simulink model "xEMU_SimulationModel3_rule1"  (R2017b)
settings: Solver=ode4  StartTime=0.0  StopTime=8192  FixedStep=0.01  RelTol=1e-3
undefined symbols (not defined in the file): a1, a2, a3, a4, ACO, BAT, Battery, DCT, DRT, EMS, ENV, Fahrzyklus_VS_modell, height_BAT, leistung, lib_bat, Maximum, Maximum_position, Num_cells, P_FC_max_long, P_FC_min_long, P_FC_step_max, Pbat_charge_max, Pbat_discharge_max, Pfc_max, Pfc_min, SOC_tar, time_peaks, TRM, velocity_peaks
libraries: simulink x5
(part 4 of 15)

== system xEMU_SimulationModel3_rule1/Battery (BAT)_komplex/Subsystem/ElectricalCircuit/Cellelement_Elem1 ==
  OhmicResistance_Elem1 : Subsystem
  ParallelRC_Elem5 : Subsystem
  ParallelRC_Elem6 : Subsystem
  Rmphn_Elem2 : Subsystem
  Rmphn_Elem3 : Subsystem
  SoC : Integrator  InitialCondition=SOC_tar*100  LimitOutput=on  UpperSaturationLimit=100  LowerSaturationLimit=0
  SoCFactor : Gain  Gain=0.001207729468599
  SphericalDiffusion_Elem4 : Subsystem
  VoltageSource_Elem7 : Subsystem
  Out1 : Outport
  wires:
  [I_CellElement1] -> SoCFactor/1
  SoCFactor/1 -> SoC/1
  [T_CellElement1] -> ParallelRC_Elem6/1(T), VoltageSource_Elem7/1(T), ParallelRC_Elem5/1(T), SphericalDiffusion_Elem4/1(T), Rmphn_Elem3/1(T), Rmphn_Elem2/1(T), OhmicResistance_Elem1/1(T)
  SoC/1 -> Out1/1, ParallelRC_Elem6/2(SoC), VoltageSource_Elem7/2(SoC), ParallelRC_Elem5/2(SoC), SphericalDiffusion_Elem4/2(SoC), Rmphn_Elem3/2(SoC), Rmphn_Elem2/2(SoC), OhmicResistance_Elem1/2(SoC)

== system xEMU_SimulationModel3_rule1/Battery (BAT)_komplex/Subsystem/MatrixAxC/StateComponent0 ==
  Add5_1 : Sum
  ColConst : Constant  Value=0
  Const1_1 : Constant  Value=-1.000000
  Const1_5 : Constant  Value=0.991746
  Const1_6 : Constant  Value=0.991451
  Const2_2 : Constant  Value=0.991451
  Div2_1 : Product  Inputs=*/
  Div2_3 : Product  Inputs=*/
  Div2_4 : Product  Inputs=*/
  Div3_2 : Product  Inputs=*/
  Integrator : Integrator
  Mul3_4 : Product
  Mul4_1 : Product
  Mul4_2 : Product
  RowConst : Constant  Value=0
  Row : Outport
  Col : Outport  Port=2
  tag scope: State1=global
  wires:
  Integrator/1 -> [State1]
  ColConst/1 -> Col/1
  RowConst/1 -> Row/1
  Add5_1/1 -> Integrator/1
  Mul4_1/1 -> Add5_1/1
  [State1] -> Mul4_1/1
  Div3_2/1 -> Mul4_1/2
  Div2_1/1 -> Div3_2/1
  Const1_1/1 -> Div2_1/1
  [ID6_ObjTau] -> Div2_1/2
  Const2_2/1 -> Div3_2/2
  Mul4_2/1 -> Add5_1/2
  [InputCurrent] -> Mul4_2/1
  Mul3_4/1 -> Mul4_2/2
  Div2_3/1 -> Mul3_4/1
  [ID6_ObjR] -> Div2_3/1
  [ID6_ObjTau] -> Div2_3/2
  Div2_4/1 -> Mul3_4/2
  Const1_5/1 -> Div2_4/1
  Const1_6/1 -> Div2_4/2

== system xEMU_SimulationModel3_rule1/Battery (BAT)_komplex/Subsystem/MatrixAxC/StateComponent1 ==
  Add5_1 : Sum
  ColConst : Constant  Value=0
  Const1_1 : Constant  Value=-1.000000
  Const1_5 : Constant  Value=0.335190
  Const1_6 : Constant  Value=0.335870
  Const2_2 : Constant  Value=0.335870
  Div2_1 : Product  Inputs=*/
  Div2_3 : Product  Inputs=*/
  Div2_4 : Product  Inputs=*/
  Div3_2 : Product  Inputs=*/
  Integrator : Integrator
  Mul3_4 : Product
  Mul4_1 : Product
  Mul4_2 : Product
  RowConst : Constant
  Row : Outport
  Col : Outport  Port=2
  tag scope: State2=global
  wires:
  Integrator/1 -> [State2]
  ColConst/1 -> Col/1
  RowConst/1 -> Row/1
  Add5_1/1 -> Integrator/1
  Mul4_1/1 -> Add5_1/1
  [State2] -> Mul4_1/1
  Div3_2/1 -> Mul4_1/2
  Div2_1/1 -> Div3_2/1
  Const1_1/1 -> Div2_1/1
  [ID6_ObjTau] -> Div2_1/2
  Const2_2/1 -> Div3_2/2
  Mul4_2/1 -> Add5_1/2
  [InputCurrent] -> Mul4_2/1
  Mul3_4/1 -> Mul4_2/2
  Div2_3/1 -> Mul3_4/1
  [ID6_ObjR] -> Div2_3/1
  [ID6_ObjTau] -> Div2_3/2
  Div2_4/1 -> Mul3_4/2
  Const1_5/1 -> Div2_4/1
  Const1_6/1 -> Div2_4/2

== system xEMU_SimulationModel3_rule1/Battery (BAT)_komplex/Subsystem/MatrixAxC/StateComponent10 ==
  Add5_1 : Sum
  ColConst : Constant  Value=0
  Const1_1 : Constant  Value=-1.000000
  Const1_5 : Constant  Value=0.020606
  Const1_6 : Constant  Value=0.004354
  Const2_2 : Constant  Value=0.004354
  Div2_1 : Product  Inputs=*/
  Div2_3 : Product  Inputs=*/
  Div2_4 : Product  Inputs=*/
  Div3_2 : Product  Inputs=*/
  Integrator : Integrator
  Mul3_4 : Product
  Mul4_1 : Product
  Mul4_2 : Product
  RowConst : Constant  Value=10
  Row : Outport
  Col : Outport  Port=2
  tag scope: State11=global
  wires:
  Integrator/1 -> [State11]
  ColConst/1 -> Col/1
  RowConst/1 -> Row/1
  Add5_1/1 -> Integrator/1
  Mul4_1/1 -> Add5_1/1
  [State11] -> Mul4_1/1
  Div3_2/1 -> Mul4_1/2
  Div2_1/1 -> Div3_2/1
  Const1_1/1 -> Div2_1/1
  [ID6_ObjTau] -> Div2_1/2
  Const2_2/1 -> Div3_2/2
  Mul4_2/1 -> Add5_1/2
  [InputCurrent] -> Mul4_2/1
  Mul3_4/1 -> Mul4_2/2
  Div2_3/1 -> Mul3_4/1
  [ID6_ObjR] -> Div2_3/1
  [ID6_ObjTau] -> Div2_3/2
  Div2_4/1 -> Mul3_4/2
  Const1_5/1 -> Div2_4/1
  Const1_6/1 -> Div2_4/2

== system xEMU_SimulationModel3_rule1/Battery (BAT)_komplex/Subsystem/MatrixAxC/StateComponent11 ==
  Add5_1 : Sum
  ColConst : Constant  Value=0
  Const1_1 : Constant  Value=-1.000000
  Const1_5 : Constant  Value=0.016393
  Const1_6 : Constant  Value=0.002781
  Const2_2 : Constant  Value=0.002781
  Div2_1 : Product  Inputs=*/
  Div2_3 : Product  Inputs=*/
  Div2_4 : Product  Inputs=*/
  Div3_2 : Product  Inputs=*/
  Integrator : Integrator
  Mul3_4 : Product
  Mul4_1 : Product
  Mul4_2 : Product
  RowConst : Constant  Value=11
  Row : Outport
  Col : Outport  Port=2
  tag scope: State12=global
  wires:
  Integrator/1 -> [State12]
  ColConst/1 -> Col/1
  RowConst/1 -> Row/1
  Add5_1/1 -> Integrator/1
  Mul4_1/1 -> Add5_1/1
  [State12] -> Mul4_1/1
  Div3_2/1 -> Mul4_1/2
  Div2_1/1 -> Div3_2/1
  Const1_1/1 -> Div2_1/1
  [ID6_ObjTau] -> Div2_1/2
  Const2_2/1 -> Div3_2/2
  Mul4_2/1 -> Add5_1/2
  [InputCurrent] -> Mul4_2/1
  Mul3_4/1 -> Mul4_2/2
  Div2_3/1 -> Mul3_4/1
  [ID6_ObjR] -> Div2_3/1
  [ID6_ObjTau] -> Div2_3/2
  Div2_4/1 -> Mul3_4/2
  Const1_5/1 -> Div2_4/1
  Const1_6/1 -> Div2_4/2

== system xEMU_SimulationModel3_rule1/Battery (BAT)_komplex/Subsystem/MatrixAxC/StateComponent12 ==
  Add5_1 : Sum
  ColConst : Constant  Value=0
  Const1_1 : Constant  Value=-1.000000
  Const1_5 : Constant  Value=0.013339
  Const1_6 : Constant  Value=0.001779
  Const2_2 : Constant  Value=0.001779
  Div2_1 : Product  Inputs=*/
  Div2_3 : Product  Inputs=*/
  Div2_4 : Product  Inputs=*/
  Div3_2 : Product  Inputs=*/
  Integrator : Integrator
  Mul3_4 : Product
  Mul4_1 : Product
  Mul4_2 : Product
  RowConst : Constant  Value=12
  Row : Outport
  Col : Outport  Port=2
  tag scope: State13=global
  wires:
  Integrator/1 -> [State13]
  ColConst/1 -> Col/1
  RowConst/1 -> Row/1
  Add5_1/1 -> Integrator/1
  Mul4_1/1 -> Add5_1/1
  [State13] -> Mul4_1/1
  Div3_2/1 -> Mul4_1/2
  Div2_1/1 -> Div3_2/1
  Const1_1/1 -> Div2_1/1
  [ID6_ObjTau] -> Div2_1/2
  Const2_2/1 -> Div3_2/2
  Mul4_2/1 -> Add5_1/2
  [InputCurrent] -> Mul4_2/1
  Mul3_4/1 -> Mul4_2/2
  Div2_3/1 -> Mul3_4/1
  [ID6_ObjR] -> Div2_3/1
  [ID6_ObjTau] -> Div2_3/2
  Div2_4/1 -> Mul3_4/2
  Const1_5/1 -> Div2_4/1
  Const1_6/1 -> Div2_4/2

== system xEMU_SimulationModel3_rule1/Battery (BAT)_komplex/Subsystem/MatrixAxC/StateComponent13 ==
  Add5_1 : Sum
  ColConst : Constant  Value=0
  Const1_1 : Constant  Value=-1.000000
  Const1_5 : Constant  Value=0.009631
  Const1_6 : Constant  Value=0.001139
  Const2_2 : Constant  Value=0.001139
  Div2_1 : Product  Inputs=*/
  Div2_3 : Product  Inputs=*/
  Div2_4 : Product  Inputs=*/
  Div3_2 : Product  Inputs=*/
  Integrator : Integrator
  Mul3_4 : Product
  Mul4_1 : Product
  Mul4_2 : Product
  RowConst : Constant  Value=13
  Row : Outport
  Col : Outport  Port=2
  tag scope: State14=global
  wires:
  Integrator/1 -> [State14]
  ColConst/1 -> Col/1
  RowConst/1 -> Row/1
  Add5_1/1 -> Integrator/1
  Mul4_1/1 -> Add5_1/1
  [State14] -> Mul4_1/1
  Div3_2/1 -> Mul4_1/2
  Div2_1/1 -> Div3_2/1
  Const1_1/1 -> Div2_1/1
  [ID6_ObjTau] -> Div2_1/2
  Const2_2/1 -> Div3_2/2
  Mul4_2/1 -> Add5_1/2
  [InputCurrent] -> Mul4_2/1
  Mul3_4/1 -> Mul4_2/2
  Div2_3/1 -> Mul3_4/1
  [ID6_ObjR] -> Div2_3/1
  [ID6_ObjTau] -> Div2_3/2
  Div2_4/1 -> Mul3_4/2
  Const1_5/1 -> Div2_4/1
  Const1_6/1 -> Div2_4/2

== system xEMU_SimulationModel3_rule1/Battery (BAT)_komplex/Subsystem/MatrixAxC/StateComponent14 ==
  Add5_1 : Sum
  ColConst : Constant  Value=0
  Const1_1 : Constant  Value=-1.000000
  Const1_5 : Constant  Value=0.010562
  Const1_6 : Constant  Value=0.000732
  Const2_2 : Constant  Value=0.000732
  Div2_1 : Product  Inputs=*/
  Div2_3 : Product  Inputs=*/
  Div2_4 : Product  Inputs=*/
  Div3_2 : Product  Inputs=*/
  Integrator : Integrator
  Mul3_4 : Product
  Mul4_1 : Product
  Mul4_2 : Product
  RowConst : Constant  Value=14
  Row : Outport
  Col : Outport  Port=2
  tag scope: State15=global
  wires:
  Integrator/1 -> [State15]
  ColConst/1 -> Col/1
  RowConst/1 -> Row/1
  Add5_1/1 -> Integrator/1
  Mul4_1/1 -> Add5_1/1
  [State15] -> Mul4_1/1
  Div3_2/1 -> Mul4_1/2
  Div2_1/1 -> Div3_2/1
  Const1_1/1 -> Div2_1/1
  [ID6_ObjTau] -> Div2_1/2
  Const2_2/1 -> Div3_2/2
  Mul4_2/1 -> Add5_1/2
  [InputCurrent] -> Mul4_2/1
  Mul3_4/1 -> Mul4_2/2
  Div2_3/1 -> Mul3_4/1
  [ID6_ObjR] -> Div2_3/1
  [ID6_ObjTau] -> Div2_3/2
  Div2_4/1 -> Mul3_4/2
  Const1_5/1 -> Div2_4/1
  Const1_6/1 -> Div2_4/2

== system xEMU_SimulationModel3_rule1/Battery (BAT)_komplex/Subsystem/MatrixAxC/StateComponent15 ==
  Add5_1 : Sum
  ColConst : Constant  Value=0
  Const1_1 : Constant  Value=-1.000000
  Const1_5 : Constant  Value=0.006255
  Const1_6 : Constant  Value=0.000468
  Const2_2 : Constant  Value=0.000468
  Div2_1 : Product  Inputs=*/
  Div2_3 : Product  Inputs=*/
  Div2_4 : Product  Inputs=*/
  Div3_2 : Product  Inputs=*/
  Integrator : Integrator
  Mul3_4 : Product
  Mul4_1 : Product
  Mul4_2 : Product
  RowConst : Constant  Value=15
  Row : Outport
  Col : Outport  Port=2
  tag scope: State16=global
  wires:
  Integrator/1 -> [State16]
  ColConst/1 -> Col/1
  RowConst/1 -> Row/1
  Add5_1/1 -> Integrator/1
  Mul4_1/1 -> Add5_1/1
  [State16] -> Mul4_1/1
  Div3_2/1 -> Mul4_1/2
  Div2_1/1 -> Div3_2/1
  Const1_1/1 -> Div2_1/1
  [ID6_ObjTau] -> Div2_1/2
  Const2_2/1 -> Div3_2/2
  Mul4_2/1 -> Add5_1/2
  [InputCurrent] -> Mul4_2/1
  Mul3_4/1 -> Mul4_2/2
  Div2_3/1 -> Mul3_4/1
  [ID6_ObjR] -> Div2_3/1
  [ID6_ObjTau] -> Div2_3/2
  Div2_4/1 -> Mul3_4/2
  Const1_5/1 -> Div2_4/1
  Const1_6/1 -> Div2_4/2

== system xEMU_SimulationModel3_rule1/Battery (BAT)_komplex/Subsystem/MatrixAxC/StateComponent16 ==
  Add5_1 : Sum
  ColConst : Constant  Value=0
  Const1_1 : Constant  Value=-1.000000
  Const1_5 : Constant  Value=0.004664
  Const1_6 : Constant  Value=0.000300
  Const2_2 : Constant  Value=0.000300
  Div2_1 : Product  Inputs=*/
  Div2_3 : Product  Inputs=*/
  Div2_4 : Product  Inputs=*/
  Div3_2 : Product  Inputs=*/
  Integrator : Integrator
  Mul3_4 : Product
  Mul4_1 : Product
  Mul4_2 : Product
  RowConst : Constant  Value=16
  Row : Outport
  Col : Outport  Port=2
  tag scope: State17=global
  wires:
  Integrator/1 -> [State17]
  ColConst/1 -> Col/1
  RowConst/1 -> Row/1
  Add5_1/1 -> Integrator/1
  Mul4_1/1 -> Add5_1/1
  [State17] -> Mul4_1/1
  Div3_2/1 -> Mul4_1/2
  Div2_1/1 -> Div3_2/1
  Const1_1/1 -> Div2_1/1
  [ID6_ObjTau] -> Div2_1/2
  Const2_2/1 -> Div3_2/2
  Mul4_2/1 -> Add5_1/2
  [InputCurrent] -> Mul4_2/1
  Mul3_4/1 -> Mul4_2/2
  Div2_3/1 -> Mul3_4/1
  [ID6_ObjR] -> Div2_3/1
  [ID6_ObjTau] -> Div2_3/2
  Div2_4/1 -> Mul3_4/2
  Const1_5/1 -> Div2_4/1
  Const1_6/1 -> Div2_4/2

== system xEMU_SimulationModel3_rule1/Battery (BAT)_komplex/Subsystem/MatrixAxC/StateComponent17 ==
  Add5_1 : Sum
  ColConst : Constant  Value=0
  Const1_1 : Constant  Value=1.000000
  Div2_1 : Product  Inputs=*/
  Div4_2 : Product  Inputs=*/
  Integrator : Integrator
  Mul3_3 : Product
  Mul4_1 : Product
  Neg3_2 : Gain  Gain=-1
  RowConst : Constant  Value=17
  Row : Outport
  Col : Outport  Port=2
  tag scope: State18=global
  wires:
  Integrator/1 -> [State18]
  ColConst/1 -> Col/1
  RowConst/1 -> Row/1
  Add5_1/1 -> Integrator/1
  Mul4_1/1 -> Add5_1/1
  [State18] -> Mul4_1/1
  Neg3_2/1 -> Mul4_1/2
  Div2_1/1 -> Neg3_2/1
  Const1_1/1 -> Div2_1/1
  [ID2_ObjTau] -> Div2_1/2
  Div4_2/1 -> Add5_1/2
  Mul3_3/1 -> Div4_2/1
  [InputCurrent] -> Mul3_3/1
  [ID2_ObjR] -> Mul3_3/2
  [ID2_ObjTau] -> Div4_2/2

== system xEMU_SimulationModel3_rule1/Battery (BAT)_komplex/Subsystem/MatrixAxC/StateComponent18 ==
  Add5_1 : Sum
  ColConst : Constant  Value=0
  Const1_1 : Constant  Value=1.000000
  Div2_1 : Product  Inputs=*/
  Div4_2 : Product  Inputs=*/
  Integrator : Integrator
  Mul3_3 : Product
  Mul4_1 : Product
  Neg3_2 : Gain  Gain=-1
  RowConst : Constant  Value=18
  Row : Outport
  Col : Outport  Port=2
  tag scope: State19=global
  wires:
  Integrator/1 -> [State19]
  ColConst/1 -> Col/1
  RowConst/1 -> Row/1
  Add5_1/1 -> Integrator/1
  Mul4_1/1 -> Add5_1/1
  [State19] -> Mul4_1/1
  Neg3_2/1 -> Mul4_1/2
  Div2_1/1 -> Neg3_2/1
  Const1_1/1 -> Div2_1/1
  [ID3_ObjTau] -> Div2_1/2
  Div4_2/1 -> Add5_1/2
  Mul3_3/1 -> Div4_2/1
  [InputCurrent] -> Mul3_3/1
  [ID3_ObjR] -> Mul3_3/2
  [ID3_ObjTau] -> Div4_2/2

== system xEMU_SimulationModel3_rule1/Battery (BAT)_komplex/Subsystem/MatrixAxC/StateComponent2 ==
  Add5_1 : Sum
  ColConst : Constant  Value=0
  Const1_1 : Constant  Value=-1.000000
  Const1_5 : Constant  Value=0.172210
  Const1_6 : Constant  Value=0.167580
  Const2_2 : Constant  Value=0.167580
  Div2_1 : Product  Inputs=*/
  Div2_3 : Product  Inputs=*/
  Div2_4 : Product  Inputs=*/
  Div3_2 : Product  Inputs=*/
  Integrator : Integrator
  Mul3_4 : Product
  Mul4_1 : Product
  Mul4_2 : Product
  RowConst : Constant  Value=2
  Row : Outport
  Col : Outport  Port=2
  tag scope: State3=global
  wires:
  Integrator/1 -> [State3]
  ColConst/1 -> Col/1
  RowConst/1 -> Row/1
  Add5_1/1 -> Integrator/1
  Mul4_1/1 -> Add5_1/1
  [State3] -> Mul4_1/1
  Div3_2/1 -> Mul4_1/2
  Div2_1/1 -> Div3_2/1
  Const1_1/1 -> Div2_1/1
  [ID6_ObjTau] -> Div2_1/2
  Const2_2/1 -> Div3_2/2
  Mul4_2/1 -> Add5_1/2
  [InputCurrent] -> Mul4_2/1
  Mul3_4/1 -> Mul4_2/2
  Div2_3/1 -> Mul3_4/1
  [ID6_ObjR] -> Div2_3/1
  [ID6_ObjTau] -> Div2_3/2
  Div2_4/1 -> Mul3_4/2
  Const1_5/1 -> Div2_4/1
  Const1_6/1 -> Div2_4/2

== system xEMU_SimulationModel3_rule1/Battery (BAT)_komplex/Subsystem/MatrixAxC/StateComponent3 ==
  Add5_1 : Sum
  ColConst : Constant  Value=0
  Const1_1 : Constant  Value=-1.000000
  Const1_5 : Constant  Value=0.099009
  Const1_6 : Constant  Value=0.097920
  Const2_2 : Constant  Value=0.097920
  Div2_1 : Product  Inputs=*/
  Div2_3 : Product  Inputs=*/
  Div2_4 : Product  Inputs=*/
  Div3_2 : Product  Inputs=*/
  Integrator : Integrator
  Mul3_4 : Product
  Mul4_1 : Product
  Mul4_2 : Product
  RowConst : Constant  Value=3
  Row : Outport
  Col : Outport  Port=2
  tag scope: State4=global
  wires:
  Integrator/1 -> [State4]
  ColConst/1 -> Col/1
  RowConst/1 -> Row/1
  Add5_1/1 -> Integrator/1
  Mul4_1/1 -> Add5_1/1
  [State4] -> Mul4_1/1
  Div3_2/1 -> Mul4_1/2
  Div2_1/1 -> Div3_2/1
  Const1_1/1 -> Div2_1/1
  [ID6_ObjTau] -> Div2_1/2
  Const2_2/1 -> Div3_2/2
  Mul4_2/1 -> Add5_1/2
  [InputCurrent] -> Mul4_2/1
  Mul3_4/1 -> Mul4_2/2
  Div2_3/1 -> Mul3_4/1
  [ID6_ObjR] -> Div2_3/1
  [ID6_ObjTau] -> Div2_3/2
  Div2_4/1 -> Mul3_4/2
  Const1_5/1 -> Div2_4/1
  Const1_6/1 -> Div2_4/2

== system xEMU_SimulationModel3_rule1/Battery (BAT)_komplex/Subsystem/MatrixAxC/StateComponent4 ==
  Add5_1 : Sum
  ColConst : Constant  Value=0
  Const1_1 : Constant  Value=-1.000000
  Const1_5 : Constant  Value=0.089432
  Const1_6 : Constant  Value=0.061684
  Const2_2 : Constant  Value=0.061684
  Div2_1 : Product  Inputs=*/
  Div2_3 : Product  Inputs=*/
  Div2_4 : Product  Inputs=*/
  Div3_2 : Product  Inputs=*/
  Integrator : Integrator
  Mul3_4 : Product
  Mul4_1 : Product
  Mul4_2 : Product
  RowConst : Constant  Value=4
  Row : Outport
  Col : Outport  Port=2
  tag scope: State5=global
  wires:
  Integrator/1 -> [State5]
  ColConst/1 -> Col/1
  RowConst/1 -> Row/1
  Add5_1/1 -> Integrator/1
  Mul4_1/1 -> Add5_1/1
  [State5] -> Mul4_1/1
  Div3_2/1 -> Mul4_1/2
  Div2_1/1 -> Div3_2/1
  Const1_1/1 -> Div2_1/1
  [ID6_ObjTau] -> Div2_1/2
  Const2_2/1 -> Div3_2/2
  Mul4_2/1 -> Add5_1/2
  [InputCurrent] -> Mul4_2/1
  Mul3_4/1 -> Mul4_2/2
  Div2_3/1 -> Mul3_4/1
  [ID6_ObjR] -> Div2_3/1
  [ID6_ObjTau] -> Div2_3/2
  Div2_4/1 -> Mul3_4/2
  Const1_5/1 -> Div2_4/1
  Const1_6/1 -> Div2_4/2

== system xEMU_SimulationModel3_rule1/Battery (BAT)_komplex/Subsystem/MatrixAxC/StateComponent5 ==
  Add5_1 : Sum
  ColConst : Constant  Value=0
  Const1_1 : Constant  Value=-1.000000
  Const1_5 : Constant  Value=0.062853
  Const1_6 : Constant  Value=0.039662
  Const2_2 : Constant  Value=0.039662
  Div2_1 : Product  Inputs=*/
  Div2_3 : Product  Inputs=*/
  Div2_4 : Product  Inputs=*/
  Div3_2 : Product  Inputs=*/
  Integrator : Integrator
  Mul3_4 : Product
  Mul4_1 : Product
  Mul4_2 : Product
  RowConst : Constant  Value=5
  Row : Outport
  Col : Outport  Port=2
  tag scope: State6=global
  wires:
  Integrator/1 -> [State6]
  ColConst/1 -> Col/1
  RowConst/1 -> Row/1
  Add5_1/1 -> Integrator/1
  Mul4_1/1 -> Add5_1/1
  [State6] -> Mul4_1/1
  Div3_2/1 -> Mul4_1/2
  Div2_1/1 -> Div3_2/1
  Const1_1/1 -> Div2_1/1
  [ID6_ObjTau] -> Div2_1/2
  Const2_2/1 -> Div3_2/2
  Mul4_2/1 -> Add5_1/2
  [InputCurrent] -> Mul4_2/1
  Mul3_4/1 -> Mul4_2/2
  Div2_3/1 -> Mul3_4/1
  [ID6_ObjR] -> Div2_3/1
  [ID6_ObjTau] -> Div2_3/2
  Div2_4/1 -> Mul3_4/2
  Const1_5/1 -> Div2_4/1
  Const1_6/1 -> Div2_4/2

== system xEMU_SimulationModel3_rule1/Battery (BAT)_komplex/Subsystem/MatrixAxC/StateComponent6 ==
  Add5_1 : Sum
  ColConst : Constant  Value=0
  Const1_1 : Constant  Value=-1.000000
  Const1_5 : Constant  Value=0.043365
  Const1_6 : Constant  Value=0.025741
  Const2_2 : Constant  Value=0.025741
  Div2_1 : Product  Inputs=*/
  Div2_3 : Product  Inputs=*/
  Div2_4 : Product  Inputs=*/
  Div3_2 : Product  Inputs=*/
  Integrator : Integrator
  Mul3_4 : Product
  Mul4_1 : Product
  Mul4_2 : Product
  RowConst : Constant  Value=6
  Row : Outport
  Col : Outport  Port=2
  tag scope: State7=global
  wires:
  Integrator/1 -> [State7]
  ColConst/1 -> Col/1
  RowConst/1 -> Row/1
  Add5_1/1 -> Integrator/1
  Mul4_1/1 -> Add5_1/1
  [State7] -> Mul4_1/1
  Div3_2/1 -> Mul4_1/2
  Div2_1/1 -> Div3_2/1
  Const1_1/1 -> Div2_1/1
  [ID6_ObjTau] -> Div2_1/2
  Const2_2/1 -> Div3_2/2
  Mul4_2/1 -> Add5_1/2
  [InputCurrent] -> Mul4_2/1
  Mul3_4/1 -> Mul4_2/2
  Div2_3/1 -> Mul3_4/1
  [ID6_ObjR] -> Div2_3/1
  [ID6_ObjTau] -> Div2_3/2
  Div2_4/1 -> Mul3_4/2
  Const1_5/1 -> Div2_4/1
  Const1_6/1 -> Div2_4/2

== system xEMU_SimulationModel3_rule1/Battery (BAT)_komplex/Subsystem/MatrixAxC/StateComponent7 ==
  Add5_1 : Sum
  ColConst : Constant  Value=0
  Const1_1 : Constant  Value=-1.000000
  Const1_5 : Constant  Value=0.040947
  Const1_6 : Constant  Value=0.016677
  Const2_2 : Constant  Value=0.016677
  Div2_1 : Product  Inputs=*/
  Div2_3 : Product  Inputs=*/
  Div2_4 : Product  Inputs=*/
  Div3_2 : Product  Inputs=*/
  Integrator : Integrator
  Mul3_4 : Product
  Mul4_1 : Product
  Mul4_2 : Product
  RowConst : Constant  Value=7
  Row : Outport
  Col : Outport  Port=2
  tag scope: State8=global
  wires:
  Integrator/1 -> [State8]
  ColConst/1 -> Col/1
  RowConst/1 -> Row/1
  Add5_1/1 -> Integrator/1
  Mul4_1/1 -> Add5_1/1
  [State8] -> Mul4_1/1
  Div3_2/1 -> Mul4_1/2
  Div2_1/1 -> Div3_2/1
  Const1_1/1 -> Div2_1/1
  [ID6_ObjTau] -> Div2_1/2
  Const2_2/1 -> Div3_2/2
  Mul4_2/1 -> Add5_1/2
  [InputCurrent] -> Mul4_2/1
  Mul3_4/1 -> Mul4_2/2
  Div2_3/1 -> Mul3_4/1
  [ID6_ObjR] -> Div2_3/1
  [ID6_ObjTau] -> Div2_3/2
  Div2_4/1 -> Mul3_4/2
  Const1_5/1 -> Div2_4/1
  Const1_6/1 -> Div2_4/2

== system xEMU_SimulationModel3_rule1/Battery (BAT)_komplex/Subsystem/MatrixAxC/StateComponent8 ==
  Add5_1 : Sum
  ColConst : Constant  Value=0
  Const1_1 : Constant  Value=-1.000000
  Const1_5 : Constant  Value=0.035960
  Const1_6 : Constant  Value=0.010685
  Const2_2 : Constant  Value=0.010685
  Div2_1 : Product  Inputs=*/
  Div2_3 : Product  Inputs=*/
  Div2_4 : Product  Inputs=*/
  Div3_2 : Product  Inputs=*/
  Integrator : Integrator
  Mul3_4 : Product
  Mul4_1 : Product
  Mul4_2 : Product
  RowConst : Constant  Value=8
  Row : Outport
  Col : Outport  Port=2
  tag scope: State9=global
  wires:
  Integrator/1 -> [State9]
  ColConst/1 -> Col/1
  RowConst/1 -> Row/1
  Add5_1/1 -> Integrator/1
  Mul4_1/1 -> Add5_1/1
  [State9] -> Mul4_1/1
  Div3_2/1 -> Mul4_1/2
  Div2_1/1 -> Div3_2/1
  Const1_1/1 -> Div2_1/1
  [ID6_ObjTau] -> Div2_1/2
  Const2_2/1 -> Div3_2/2
  Mul4_2/1 -> Add5_1/2
  [InputCurrent] -> Mul4_2/1
  Mul3_4/1 -> Mul4_2/2
  Div2_3/1 -> Mul3_4/1
  [ID6_ObjR] -> Div2_3/1
  [ID6_ObjTau] -> Div2_3/2
  Div2_4/1 -> Mul3_4/2
  Const1_5/1 -> Div2_4/1
  Const1_6/1 -> Div2_4/2

== system xEMU_SimulationModel3_rule1/Battery (BAT)_komplex/Subsystem/MatrixAxC/StateComponent9 ==
  Add5_1 : Sum
  ColConst : Constant  Value=0
  Const1_1 : Constant  Value=-1.000000
  Const1_5 : Constant  Value=0.025709
  Const1_6 : Constant  Value=0.006818
  Const2_2 : Constant  Value=0.006818
  Div2_1 : Product  Inputs=*/
  Div2_3 : Product  Inputs=*/
  Div2_4 : Product  Inputs=*/
  Div3_2 : Product  Inputs=*/
  Integrator : Integrator
  Mul3_4 : Product
  Mul4_1 : Product
  Mul4_2 : Product
  RowConst : Constant  Value=9
  Row : Outport
  Col : Outport  Port=2
  tag scope: State10=global
  wires:
  Integrator/1 -> [State10]
  ColConst/1 -> Col/1
  RowConst/1 -> Row/1
  Add5_1/1 -> Integrator/1
  Mul4_1/1 -> Add5_1/1
  [State10] -> Mul4_1/1
  Div3_2/1 -> Mul4_1/2
  Div2_1/1 -> Div3_2/1
  Const1_1/1 -> Div2_1/1
  [ID6_ObjTau] -> Div2_1/2
  Const2_2/1 -> Div3_2/2
  Mul4_2/1 -> Add5_1/2
  [InputCurrent] -> Mul4_2/1
  Mul3_4/1 -> Mul4_2/2
  Div2_3/1 -> Mul3_4/1
  [ID6_ObjR] -> Div2_3/1
  [ID6_ObjTau] -> Div2_3/2
  Div2_4/1 -> Mul3_4/2
  Const1_5/1 -> Div2_4/1
  Const1_6/1 -> Div2_4/2

== system xEMU_SimulationModel3_rule1/Battery (BAT)_komplex/Subsystem/PowerMatrix/Component0 ==
  Add4_1 : Sum
  Add5_1 : Sum
  Add6_1 : Sum
  Add7_1 : Sum
  ColConst : Constant  Value=0
  Div5_2 : Product  Inputs=*/
  Div6_2 : Product  Inputs=*/
  Mul3_1 : Product
  Mul3_2 : Product
  Mul4_2 : Product
  RowConst : Constant  Value=0
  Squ2_1 : Math  Operator=square  SaturateOnIntegerOverflow=on
  Squ2_3 : Math  Operator=square  SaturateOnIntegerOverflow=on
  Squ3_3 : Math  Operator=square  SaturateOnIntegerOverflow=on
  Squ4_3 : Math  Operator=square  SaturateOnIntegerOverflow=on
  Squ5_3 : Math  Operator=square  SaturateOnIntegerOverflow=on
  Row : Outport
  Col : Outport  Port=2
  Value : Outport  Port=3
  wires:
  ColConst/1 -> Col/1
  RowConst/1 -> Row/1
  Add7_1/1 -> Value/1
  Add6_1/1 -> Add7_1/1
  Add5_1/1 -> Add6_1/1
  Add4_1/1 -> Add5_1/1
  Mul3_1/1 -> Add4_1/1
  Squ2_1/1 -> Mul3_1/1
  [InputCurrent] -> Squ2_1/1
  [ID1_ObjR] -> Mul3_1/2
  Mul3_2/1 -> Add4_1/2
  Squ2_3/1 -> Mul3_2/1
  [InputCurrent] -> Squ2_3/1
  [ID0_ObjR] -> Mul3_2/2
  Mul4_2/1 -> Add5_1/2
  Squ3_3/1 -> Mul4_2/1
  [InputCurrent] -> Squ3_3/1
  [ID0_ObjR] -> Mul4_2/2
  Div5_2/1 -> Add6_1/2
  Squ4_3/1 -> Div5_2/1
  [State18] -> Squ4_3/1
  [ID2_ObjR] -> Div5_2/2
  Div6_2/1 -> Add7_1/2
  Squ5_3/1 -> Div6_2/1
  [State19] -> Squ5_3/1
  [ID3_ObjR] -> Div6_2/2

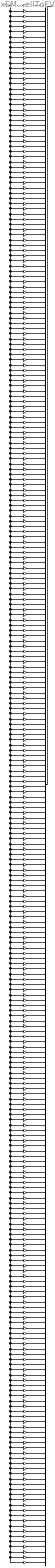
== system xEMU_SimulationModel3_rule1/Battery (BAT)_komplex/Subsystem/Thermal/CellToFV ==
  Mux : Mux  Inputs=300
  P_FV_{1..300} (300 alike) : Gain  Gain=0.0033333  SaturateOnIntegerOverflow=on  OutDataTypeStr=Inherit: Same as input  ParamDataTypeStr=Inherit: Same as input
  P_FV : Outport
  wires:
  Mux/1 -> P_FV/1
  [P_CellElement1] -> P_FV_299/1, P_FV_300/1, P_FV_298/1, P_FV_297/1, P_FV_296/1, P_FV_295/1, P_FV_294/1, P_FV_293/1, P_FV_292/1, P_FV_291/1, P_FV_290/1, P_FV_289/1, P_FV_288/1, P_FV_287/1, P_FV_286/1, P_FV_285/1, P_FV_284/1, P_FV_283/1, P_FV_282/1, P_FV_281/1, P_FV_280/1, P_FV_279/1, P_FV_278/1, P_FV_277/1, P_FV_276/1, P_FV_275/1, P_FV_274/1, P_FV_273/1, P_FV_272/1, P_FV_271/1, P_FV_270/1, P_FV_269/1, P_FV_268/1, P_FV_267/1, P_FV_266/1, P_FV_265/1, P_FV_264/1, P_FV_263/1, P_FV_262/1, P_FV_261/1, P_FV_260/1, P_FV_259/1, P_FV_258/1, P_FV_257/1, P_FV_256/1, P_FV_255/1, P_FV_254/1, P_FV_253/1, P_FV_252/1, P_FV_251/1, P_FV_250/1, P_FV_249/1, P_FV_248/1, P_FV_247/1, P_FV_246/1, P_FV_245/1, P_FV_244/1, P_FV_243/1, P_FV_242/1, P_FV_241/1, P_FV_240/1, P_FV_239/1, P_FV_238/1, P_FV_237/1, P_FV_236/1, P_FV_235/1, P_FV_234/1, P_FV_233/1, P_FV_232/1, P_FV_231/1, P_FV_230/1, P_FV_229/1, P_FV_228/1, P_FV_227/1, P_FV_226/1, P_FV_225/1, P_FV_224/1, P_FV_223/1, P_FV_222/1, P_FV_221/1, P_FV_220/1, P_FV_219/1, P_FV_218/1, P_FV_217/1, P_FV_216/1, P_FV_215/1, P_FV_214/1, P_FV_213/1, P_FV_212/1, P_FV_211/1, P_FV_210/1, P_FV_209/1, P_FV_208/1, P_FV_207/1, P_FV_206/1, P_FV_205/1, P_FV_204/1, P_FV_203/1, P_FV_202/1, P_FV_201/1, P_FV_200/1, P_FV_199/1, P_FV_198/1, P_FV_197/1, P_FV_196/1, P_FV_195/1, P_FV_194/1, P_FV_193/1, P_FV_192/1, P_FV_191/1, P_FV_190/1, P_FV_189/1, P_FV_188/1, P_FV_187/1, P_FV_186/1, P_FV_185/1, P_FV_184/1, P_FV_183/1, P_FV_182/1, P_FV_181/1, P_FV_180/1, P_FV_179/1, P_FV_178/1, P_FV_177/1, P_FV_176/1, P_FV_175/1, P_FV_174/1, P_FV_173/1, P_FV_172/1, P_FV_171/1, P_FV_170/1, P_FV_169/1, P_FV_168/1, P_FV_167/1, P_FV_166/1, P_FV_165/1, P_FV_164/1, P_FV_163/1, P_FV_162/1, P_FV_161/1, P_FV_160/1, P_FV_159/1, P_FV_158/1, P_FV_157/1, P_FV_156/1, P_FV_155/1, P_FV_154/1, P_FV_153/1, P_FV_152/1, P_FV_151/1, P_FV_150/1, P_FV_149/1, P_FV_148/1, P_FV_147/1, P_FV_146/1, P_FV_145/1, P_FV_144/1, P_FV_143/1, P_FV_142/1, P_FV_141/1, P_FV_140/1, P_FV_139/1, P_FV_138/1, P_FV_137/1, P_FV_136/1, P_FV_135/1, P_FV_134/1, P_FV_133/1, P_FV_132/1, P_FV_131/1, P_FV_130/1, P_FV_129/1, P_FV_128/1, P_FV_127/1, P_FV_126/1, P_FV_125/1, P_FV_124/1, P_FV_123/1, P_FV_122/1, P_FV_121/1, P_FV_120/1, P_FV_119/1, P_FV_118/1, P_FV_117/1, P_FV_116/1, P_FV_115/1, P_FV_114/1, P_FV_113/1, P_FV_112/1, P_FV_111/1, P_FV_110/1, P_FV_109/1, P_FV_108/1, P_FV_107/1, P_FV_106/1, P_FV_105/1, P_FV_104/1, P_FV_103/1, P_FV_102/1, P_FV_101/1, P_FV_100/1, P_FV_99/1, P_FV_98/1, P_FV_97/1, P_FV_96/1, P_FV_95/1, P_FV_94/1, P_FV_93/1, P_FV_92/1, P_FV_91/1, P_FV_90/1, P_FV_89/1, P_FV_88/1, P_FV_87/1, P_FV_86/1, P_FV_85/1, P_FV_84/1, P_FV_83/1, P_FV_82/1, P_FV_81/1, P_FV_80/1, P_FV_79/1, P_FV_78/1, P_FV_77/1, P_FV_76/1, P_FV_75/1, P_FV_74/1, P_FV_73/1, P_FV_72/1, P_FV_71/1, P_FV_70/1, P_FV_69/1, P_FV_68/1, P_FV_67/1, P_FV_66/1, P_FV_65/1, P_FV_64/1, P_FV_63/1, P_FV_62/1, P_FV_61/1, P_FV_60/1, P_FV_59/1, P_FV_58/1, P_FV_57/1, P_FV_56/1, P_FV_55/1, P_FV_54/1, P_FV_53/1, P_FV_52/1, P_FV_51/1, P_FV_50/1, P_FV_49/1, P_FV_48/1, P_FV_47/1, P_FV_46/1, P_FV_45/1, P_FV_44/1, P_FV_43/1, P_FV_42/1, P_FV_41/1, P_FV_40/1, P_FV_39/1, P_FV_38/1, P_FV_37/1, P_FV_36/1, P_FV_35/1, P_FV_34/1, P_FV_33/1, P_FV_32/1, P_FV_31/1, P_FV_30/1, P_FV_29/1, P_FV_28/1, P_FV_27/1, P_FV_26/1, P_FV_25/1, P_FV_24/1, P_FV_23/1, P_FV_22/1, P_FV_21/1, P_FV_20/1, P_FV_19/1, P_FV_18/1, P_FV_17/1, P_FV_16/1, P_FV_15/1, P_FV_14/1, P_FV_13/1, P_FV_12/1, P_FV_11/1, P_FV_10/1, P_FV_9/1, P_FV_8/1, P_FV_7/1, P_FV_6/1, P_FV_5/1, P_FV_4/1, P_FV_3/1, P_FV_2/1, P_FV_1/1
  P_FV_1/1 -> Mux/1
  P_FV_2/1 -> Mux/2
  P_FV_3/1 -> Mux/3
  P_FV_4/1 -> Mux/4
  P_FV_5/1 -> Mux/5
  P_FV_6/1 -> Mux/6
  P_FV_7/1 -> Mux/7
  P_FV_8/1 -> Mux/8
  P_FV_9/1 -> Mux/9
  P_FV_10/1 -> Mux/10
  P_FV_11/1 -> Mux/11
  P_FV_12/1 -> Mux/12
  P_FV_13/1 -> Mux/13
  P_FV_14/1 -> Mux/14
  P_FV_15/1 -> Mux/15
  P_FV_16/1 -> Mux/16
  P_FV_17/1 -> Mux/17
  P_FV_18/1 -> Mux/18
  P_FV_19/1 -> Mux/19
  P_FV_20/1 -> Mux/20
  P_FV_21/1 -> Mux/21
  P_FV_22/1 -> Mux/22
  P_FV_23/1 -> Mux/23
  P_FV_24/1 -> Mux/24
  P_FV_25/1 -> Mux/25
  P_FV_26/1 -> Mux/26
  P_FV_27/1 -> Mux/27
  P_FV_28/1 -> Mux/28
  P_FV_29/1 -> Mux/29
  P_FV_30/1 -> Mux/30
  P_FV_31/1 -> Mux/31
  P_FV_32/1 -> Mux/32
  P_FV_33/1 -> Mux/33
  P_FV_34/1 -> Mux/34
  P_FV_35/1 -> Mux/35
  P_FV_36/1 -> Mux/36
  P_FV_37/1 -> Mux/37
  P_FV_38/1 -> Mux/38
  P_FV_39/1 -> Mux/39
  P_FV_40/1 -> Mux/40
  P_FV_41/1 -> Mux/41
  P_FV_42/1 -> Mux/42
  P_FV_43/1 -> Mux/43
  P_FV_44/1 -> Mux/44
  P_FV_45/1 -> Mux/45
  P_FV_46/1 -> Mux/46
  P_FV_47/1 -> Mux/47
  P_FV_48/1 -> Mux/48
  P_FV_49/1 -> Mux/49
  P_FV_50/1 -> Mux/50
  P_FV_51/1 -> Mux/51
  P_FV_52/1 -> Mux/52
  P_FV_53/1 -> Mux/53
  P_FV_54/1 -> Mux/54
  P_FV_55/1 -> Mux/55
  P_FV_56/1 -> Mux/56
  P_FV_57/1 -> Mux/57
  P_FV_58/1 -> Mux/58
  P_FV_59/1 -> Mux/59
  P_FV_60/1 -> Mux/60
  P_FV_61/1 -> Mux/61
  P_FV_62/1 -> Mux/62
  P_FV_63/1 -> Mux/63
  P_FV_64/1 -> Mux/64
  P_FV_65/1 -> Mux/65
  P_FV_66/1 -> Mux/66
  P_FV_67/1 -> Mux/67
  P_FV_68/1 -> Mux/68
  P_FV_69/1 -> Mux/69
  P_FV_70/1 -> Mux/70
  P_FV_71/1 -> Mux/71
  P_FV_72/1 -> Mux/72
  P_FV_73/1 -> Mux/73
  P_FV_74/1 -> Mux/74
  P_FV_75/1 -> Mux/75
  P_FV_76/1 -> Mux/76
  P_FV_77/1 -> Mux/77
  P_FV_78/1 -> Mux/78
  P_FV_79/1 -> Mux/79
  P_FV_80/1 -> Mux/80
  P_FV_81/1 -> Mux/81
  P_FV_82/1 -> Mux/82
  P_FV_83/1 -> Mux/83
  P_FV_84/1 -> Mux/84
  P_FV_85/1 -> Mux/85
  P_FV_86/1 -> Mux/86
  P_FV_87/1 -> Mux/87
  P_FV_88/1 -> Mux/88
  P_FV_89/1 -> Mux/89
  P_FV_90/1 -> Mux/90
  P_FV_91/1 -> Mux/91
  P_FV_92/1 -> Mux/92
  P_FV_93/1 -> Mux/93
  P_FV_94/1 -> Mux/94
  P_FV_95/1 -> Mux/95
  P_FV_96/1 -> Mux/96
  P_FV_97/1 -> Mux/97
  P_FV_98/1 -> Mux/98
  P_FV_99/1 -> Mux/99
  P_FV_100/1 -> Mux/100
  P_FV_101/1 -> Mux/101
  P_FV_102/1 -> Mux/102
  P_FV_103/1 -> Mux/103
  P_FV_104/1 -> Mux/104
  P_FV_105/1 -> Mux/105
  P_FV_106/1 -> Mux/106
  P_FV_107/1 -> Mux/107
  P_FV_108/1 -> Mux/108
  P_FV_109/1 -> Mux/109
  P_FV_110/1 -> Mux/110
  P_FV_111/1 -> Mux/111
  P_FV_112/1 -> Mux/112
  P_FV_113/1 -> Mux/113
  P_FV_114/1 -> Mux/114
  P_FV_115/1 -> Mux/115
  P_FV_116/1 -> Mux/116
  P_FV_117/1 -> Mux/117
  P_FV_118/1 -> Mux/118
  P_FV_119/1 -> Mux/119
  P_FV_120/1 -> Mux/120
  P_FV_121/1 -> Mux/121
  P_FV_122/1 -> Mux/122
  P_FV_123/1 -> Mux/123
  P_FV_124/1 -> Mux/124
  P_FV_125/1 -> Mux/125
  P_FV_126/1 -> Mux/126
  P_FV_127/1 -> Mux/127
  P_FV_128/1 -> Mux/128
  P_FV_129/1 -> Mux/129
  P_FV_130/1 -> Mux/130
  P_FV_131/1 -> Mux/131
  P_FV_132/1 -> Mux/132
  P_FV_133/1 -> Mux/133
  P_FV_134/1 -> Mux/134
  P_FV_135/1 -> Mux/135
  P_FV_136/1 -> Mux/136
  P_FV_137/1 -> Mux/137
  P_FV_138/1 -> Mux/138
  P_FV_139/1 -> Mux/139
  P_FV_140/1 -> Mux/140
  P_FV_141/1 -> Mux/141
  P_FV_142/1 -> Mux/142
  P_FV_143/1 -> Mux/143
  P_FV_144/1 -> Mux/144
  P_FV_145/1 -> Mux/145
  P_FV_146/1 -> Mux/146
  P_FV_147/1 -> Mux/147
  P_FV_148/1 -> Mux/148
  P_FV_149/1 -> Mux/149
  P_FV_150/1 -> Mux/150
  P_FV_151/1 -> Mux/151
  P_FV_152/1 -> Mux/152
  P_FV_153/1 -> Mux/153
  P_FV_154/1 -> Mux/154
  P_FV_155/1 -> Mux/155
  P_FV_156/1 -> Mux/156
  P_FV_157/1 -> Mux/157
  P_FV_158/1 -> Mux/158
  P_FV_159/1 -> Mux/159
  P_FV_160/1 -> Mux/160
  P_FV_161/1 -> Mux/161
  P_FV_162/1 -> Mux/162
  P_FV_163/1 -> Mux/163
  P_FV_164/1 -> Mux/164
  P_FV_165/1 -> Mux/165
  P_FV_166/1 -> Mux/166
  P_FV_167/1 -> Mux/167
  P_FV_168/1 -> Mux/168
  P_FV_169/1 -> Mux/169
  P_FV_170/1 -> Mux/170
  P_FV_171/1 -> Mux/171
  P_FV_172/1 -> Mux/172
  P_FV_173/1 -> Mux/173
  P_FV_174/1 -> Mux/174
  P_FV_175/1 -> Mux/175
  P_FV_176/1 -> Mux/176
  P_FV_177/1 -> Mux/177
  P_FV_178/1 -> Mux/178
  P_FV_179/1 -> Mux/179
  P_FV_180/1 -> Mux/180
  P_FV_181/1 -> Mux/181
  P_FV_182/1 -> Mux/182
  P_FV_183/1 -> Mux/183
  P_FV_184/1 -> Mux/184
  P_FV_185/1 -> Mux/185
  P_FV_186/1 -> Mux/186
  P_FV_187/1 -> Mux/187
  P_FV_188/1 -> Mux/188
  P_FV_189/1 -> Mux/189
  P_FV_190/1 -> Mux/190
  P_FV_191/1 -> Mux/191
  P_FV_192/1 -> Mux/192
  P_FV_193/1 -> Mux/193
  P_FV_194/1 -> Mux/194
  P_FV_195/1 -> Mux/195
  P_FV_196/1 -> Mux/196
  P_FV_197/1 -> Mux/197
  P_FV_198/1 -> Mux/198
  P_FV_199/1 -> Mux/199
  P_FV_200/1 -> Mux/200
  P_FV_201/1 -> Mux/201
  P_FV_202/1 -> Mux/202
  P_FV_203/1 -> Mux/203
  P_FV_204/1 -> Mux/204
  P_FV_205/1 -> Mux/205
  P_FV_206/1 -> Mux/206
  P_FV_207/1 -> Mux/207
  P_FV_208/1 -> Mux/208
  P_FV_209/1 -> Mux/209
  P_FV_210/1 -> Mux/210
  P_FV_211/1 -> Mux/211
  P_FV_212/1 -> Mux/212
  P_FV_213/1 -> Mux/213
  P_FV_214/1 -> Mux/214
  P_FV_215/1 -> Mux/215
  P_FV_216/1 -> Mux/216
  P_FV_217/1 -> Mux/217
  P_FV_218/1 -> Mux/218
  P_FV_219/1 -> Mux/219
  P_FV_220/1 -> Mux/220
  P_FV_221/1 -> Mux/221
  P_FV_222/1 -> Mux/222
  P_FV_223/1 -> Mux/223
  P_FV_224/1 -> Mux/224
  P_FV_225/1 -> Mux/225
  P_FV_226/1 -> Mux/226
  P_FV_227/1 -> Mux/227
  P_FV_228/1 -> Mux/228
  P_FV_229/1 -> Mux/229
  P_FV_230/1 -> Mux/230
  P_FV_231/1 -> Mux/231
  P_FV_232/1 -> Mux/232
  P_FV_233/1 -> Mux/233
  P_FV_234/1 -> Mux/234
  P_FV_235/1 -> Mux/235
  P_FV_236/1 -> Mux/236
  P_FV_237/1 -> Mux/237
  P_FV_238/1 -> Mux/238
  P_FV_239/1 -> Mux/239
  P_FV_240/1 -> Mux/240
  P_FV_241/1 -> Mux/241
  P_FV_242/1 -> Mux/242
  P_FV_243/1 -> Mux/243
  P_FV_244/1 -> Mux/244
  P_FV_245/1 -> Mux/245
  P_FV_246/1 -> Mux/246
  P_FV_247/1 -> Mux/247
  P_FV_248/1 -> Mux/248
  P_FV_249/1 -> Mux/249
  P_FV_250/1 -> Mux/250
  P_FV_251/1 -> Mux/251
  P_FV_252/1 -> Mux/252
  P_FV_253/1 -> Mux/253
  P_FV_254/1 -> Mux/254
  P_FV_255/1 -> Mux/255
  P_FV_256/1 -> Mux/256
  P_FV_257/1 -> Mux/257
  P_FV_258/1 -> Mux/258
  P_FV_259/1 -> Mux/259
  P_FV_260/1 -> Mux/260
  P_FV_261/1 -> Mux/261
  P_FV_262/1 -> Mux/262
  P_FV_263/1 -> Mux/263
  P_FV_264/1 -> Mux/264
  P_FV_265/1 -> Mux/265
  P_FV_266/1 -> Mux/266
  P_FV_267/1 -> Mux/267
  P_FV_268/1 -> Mux/268
  P_FV_269/1 -> Mux/269
  P_FV_270/1 -> Mux/270
  P_FV_271/1 -> Mux/271
  P_FV_272/1 -> Mux/272
  P_FV_273/1 -> Mux/273
  P_FV_274/1 -> Mux/274
  P_FV_275/1 -> Mux/275
  P_FV_276/1 -> Mux/276
  P_FV_277/1 -> Mux/277
  P_FV_278/1 -> Mux/278
  P_FV_279/1 -> Mux/279
  P_FV_280/1 -> Mux/280
  P_FV_281/1 -> Mux/281
  P_FV_282/1 -> Mux/282
  P_FV_283/1 -> Mux/283
  P_FV_284/1 -> Mux/284
  P_FV_285/1 -> Mux/285
  P_FV_286/1 -> Mux/286
  P_FV_287/1 -> Mux/287
  P_FV_288/1 -> Mux/288
  P_FV_289/1 -> Mux/289
  P_FV_290/1 -> Mux/290
  P_FV_291/1 -> Mux/291
  P_FV_292/1 -> Mux/292
  P_FV_293/1 -> Mux/293
  P_FV_294/1 -> Mux/294
  P_FV_295/1 -> Mux/295
  P_FV_296/1 -> Mux/296
  P_FV_297/1 -> Mux/297
  P_FV_298/1 -> Mux/298
  P_FV_299/1 -> Mux/299
  P_FV_300/1 -> Mux/300

== system xEMU_SimulationModel3_rule1/Battery (BAT)_komplex/Subsystem/Thermal/Coolings ==
  T_FV : Inport
  CoolAdder : Subsystem
  P_FV : Outport
  wires:
  CoolAdder/1(P_FV) -> P_FV/1
